simulink model "InductionMachine_dq"  (R2021b)
settings: Solver=FixedStepAuto  StartTime=0.0  StopTime=5  FixedStep=1e-3  RelTol=1e-3
values from neighbouring files (symbols this model uses):
  i_mr_0 = fl_rd_0 / L0    [InductionMachine_dq_cal.m]
  i_sd_0 = Isd_0    [InductionMachine_dq_cal.m]
  i_sq_0 = Isq_0    [InductionMachine_dq_cal.m]
  J = 0.2    [InductionMachine_cal.m]    (also in InductionMachine_dq_cal.m)
  L1 = 135.6e-3    (= 0.1356)    [InductionMachine_cal.m]    (also in InductionMachine_dq_cal.m)
  omega_m_0 = (2/P)*Wm    (= 188.495559215)    [InductionMachine_dq_cal.m]
  omega_vin = 120 * pi    (= 376.991118431)    [InductionMachine_dq_cal.m]
  P = 4    [InductionMachine_cal.m]    (also in InductionMachine_dq_cal.m)
  R1 = .75    (= 0.75)    [InductionMachine_cal.m]    (also in InductionMachine_dq_cal.m)
  sigma = 1 - (L0^2)/(L1*L2)    (= 0.0205423725864)    [InductionMachine_dq_cal.m]
  theta_0 = thetar    [InductionMachine_dq_cal.m]
  Tl = 0    [InductionMachine_cal.m]    (also in InductionMachine_dq_cal.m)
  Tr = L2/R2    (= 0.294782608696)    [InductionMachine_dq_cal.m]
  V_in = 163    [InductionMachine_dq_cal.m]
Description:
  | Lecture #20. page 138
  | Model of induction machine: Rotor Flux Oriented
  | Reference frame
settings Model: Creator=Dinh-Tuyen Le  LastModifiedBy=Dinh-Tuyen Le

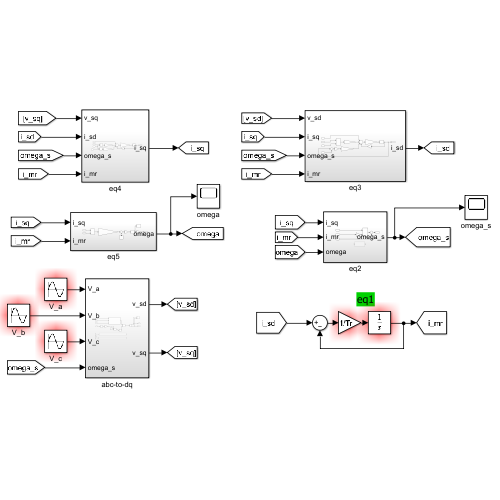
[thumbnail: Simulink's stored preview of the top-level diagram]
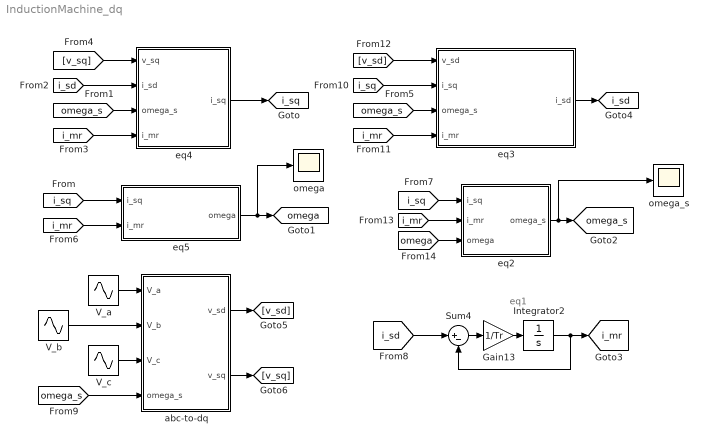
== system InductionMachine_dq ==
  note: eq1
  Gain13 : Gain  Gain=1/Tr
  Integrator2 : Integrator  InitialCondition=i_mr_0
  Sum4 : Sum  Inputs=|+-
  V_a : Sin  Amplitude=V_in  Frequency=omega_vin  Phase=pi/2  SampleTime=0
  V_b : Sin  Amplitude=V_in  Frequency=omega_vin  Phase=pi/2 -2 * pi / 3  SampleTime=0
  V_c : Sin  Amplitude=V_in  Frequency=omega_vin  Phase=pi/2 -4 * pi /3  SampleTime=0
  abc-to-dq : Subsystem
  eq2 : Subsystem
  eq3 : Subsystem
  eq4 : Subsystem
  eq5 : Subsystem
  omega : Scope
  omega_s : Scope
  tag scope: i_mr=global, i_sd=global, i_sq=global, omega=global, omega_s=global
  wires:
  [i_sd] -> Sum4/1
  Integrator2/1 -> Sum4/2, [i_mr]
  Sum4/1 -> Gain13/1
  Gain13/1 -> Integrator2/1
  V_a/1 -> abc-to-dq/1(V_a)
  V_b/1 -> abc-to-dq/2(V_b)
  V_c/1 -> abc-to-dq/3(V_c)
  [omega_s] -> abc-to-dq/4(omega_s)
  abc-to-dq/1(v_sd) -> [v_sd]
  abc-to-dq/2(v_sq) -> [v_sq]
  [i_sq] -> eq2/1(i_sq)
  [i_mr] -> eq2/2(i_mr)
  [omega] -> eq2/3(omega)
  eq2/1(omega_s) -> omega_s/1, [omega_s]
  [v_sd] -> eq3/1(v_sd)
  [i_sq] -> eq3/2(i_sq)
  [omega_s] -> eq3/3(omega_s)
  [i_mr] -> eq3/4(i_mr)
  eq3/1(i_sd) -> [i_sd]
  [i_sq] -> eq5/1(i_sq)
  [i_mr] -> eq5/2(i_mr)
  eq5/1(omega) -> omega/1, [omega]
  [v_sq] -> eq4/1(v_sq)
  [i_sd] -> eq4/2(i_sd)
  [omega_s] -> eq4/3(omega_s)
  [i_mr] -> eq4/4(i_mr)
  eq4/1(i_sq) -> [i_sq]

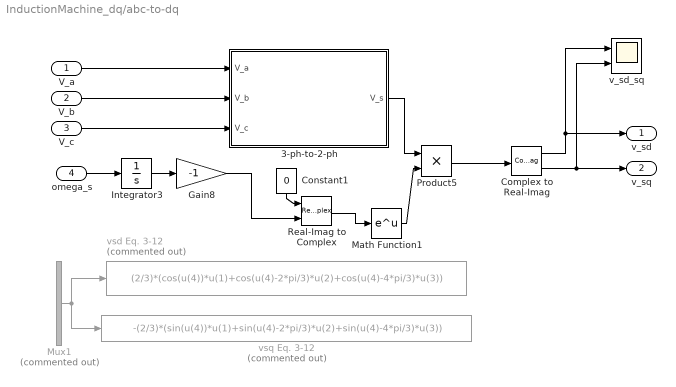
== system InductionMachine_dq/abc-to-dq ==
  V_a : Inport
  V_b : Inport  Port=2
  V_c : Inport  Port=3
  omega_s : Inport  Port=4
  3-ph-to-2-ph : Subsystem
  Complex to Real-Imag : ComplexToRealImag
  Constant1 : Constant  Value=0
  Gain8 : Gain  Gain=-1
  Integrator3 : Integrator  InitialCondition=theta_0
  Math Function1 : Math  OutputSignalType=complex  SaturateOnIntegerOverflow=on
  Mux1 : Mux  Commented=on
  Product5 : Product
  Real-Imag to Complex : RealImagToComplex
  v_sd_sq : Scope  NumInputPorts=2
  vsd Eq. 3-12 : Fcn  Commented=on  Expr=(2/3)*(cos(u(4))*u(1)+cos(u(4)-2*pi/3)*u(2)+cos(u(4)-4*pi/3)*u(3))
  vsq Eq. 3-12 : Fcn  Commented=on  Expr=-(2/3)*(sin(u(4))*u(1)+sin(u(4)-2*pi/3)*u(2)+sin(u(4)-4*pi/3)*u(3))
  v_sd : Outport
  v_sq : Outport  Port=2
  wires:
  3-ph-to-2-ph/1(V_s) -> Product5/1
  Math Function1/1 -> Product5/2
  Gain8/1 -> Real-Imag to Complex/2
  Constant1/1 -> Real-Imag to Complex/1
  Mux1/1 -> vsq Eq. 3-12/1, vsd Eq. 3-12/1
  Complex to Real-Imag/1 -> v_sd_sq/1, v_sd/1
  Real-Imag to Complex/1 -> Math Function1/1
  Integrator3/1 -> Gain8/1
  V_c/1 -> 3-ph-to-2-ph/3(V_c)
  V_b/1 -> 3-ph-to-2-ph/2(V_b)
  V_a/1 -> 3-ph-to-2-ph/1(V_a)
  omega_s/1 -> Integrator3/1
  Product5/1 -> Complex to Real-Imag/1
  Complex to Real-Imag/2 -> v_sd_sq/2, v_sq/1

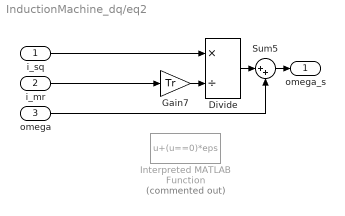
== system InductionMachine_dq/eq2 ==
  i_sq : Inport
  i_mr : Inport  Port=2
  omega : Inport  Port=3
  Divide : Product  Inputs=*/
  Gain7 : Gain  Gain=Tr
  Interpreted MATLAB Function : MATLABFcn  Commented=on  MATLABFcn=u+(u==0)*eps
  Sum5 : Sum  Inputs=|++
  omega_s : Outport
  wires:
  i_mr/1 -> Gain7/1
  Sum5/1 -> omega_s/1
  omega/1 -> Sum5/2
  Divide/1 -> Sum5/1
  i_sq/1 -> Divide/1
  Gain7/1 -> Divide/2

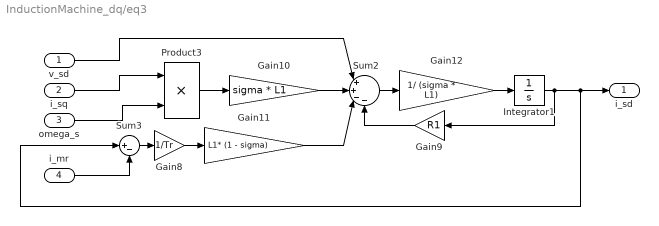
== system InductionMachine_dq/eq3 ==
  v_sd : Inport
  i_sq : Inport  Port=2
  omega_s : Inport  Port=3
  i_mr : Inport  Port=4
  Gain10 : Gain  Gain=sigma * L1
  Gain11 : Gain  Gain=L1* (1 - sigma)
  Gain12 : Gain  Gain=1/ (sigma * L1)
  Gain8 : Gain  Gain=1/Tr
  Gain9 : Gain  Gain=R1
  Integrator1 : Integrator  InitialCondition=i_sd_0
  Product3 : Product
  Sum2 : Sum  Inputs=|++--
  Sum3 : Sum  Inputs=|+-
  i_sd : Outport
  wires:
  Gain11/1 -> Sum2/3
  Sum2/1 -> Gain12/1
  i_mr/1 -> Sum3/2
  Product3/1 -> Gain10/1
  Gain10/1 -> Sum2/2
  v_sd/1 -> Sum2/1
  Integrator1/1 -> Sum3/1, i_sd/1, Gain9/1
  Gain9/1 -> Sum2/4
  Sum3/1 -> Gain8/1
  omega_s/1 -> Product3/2
  Gain8/1 -> Gain11/1
  i_sq/1 -> Product3/1
  Gain12/1 -> Integrator1/1

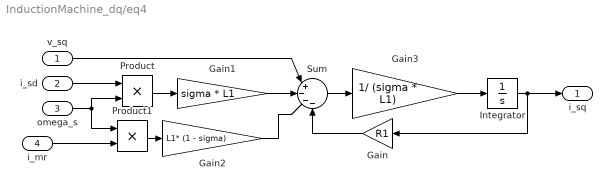
== system InductionMachine_dq/eq4 ==
  v_sq : Inport
  i_sd : Inport  Port=2
  omega_s : Inport  Port=3
  i_mr : Inport  Port=4
  Gain : Gain  Gain=R1
  Gain1 : Gain  Gain=sigma * L1
  Gain2 : Gain  Gain=L1* (1 - sigma)
  Gain3 : Gain  Gain=1/ (sigma * L1)
  Integrator : Integrator  InitialCondition=i_sq_0
  Product : Product
  Product1 : Product
  Sum : Sum  Inputs=|+---
  i_sq : Outport
  wires:
  Integrator/1 -> i_sq/1, Gain/1
  Gain1/1 -> Sum/2
  Sum/1 -> Gain3/1
  Gain3/1 -> Integrator/1
  omega_s/1 -> Product/2, Product1/1
  Gain/1 -> Sum/4
  Gain2/1 -> Sum/3
  Product1/1 -> Gain2/1
  Product/1 -> Gain1/1
  i_sd/1 -> Product/1
  v_sq/1 -> Sum/1
  i_mr/1 -> Product1/2

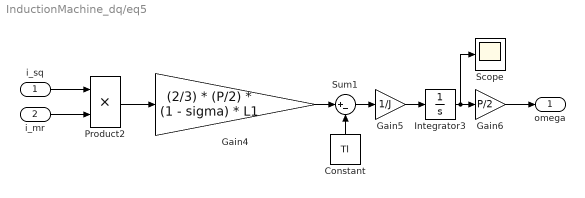
== system InductionMachine_dq/eq5 ==
  i_sq : Inport
  i_mr : Inport  Port=2
  Constant : Constant  Value=Tl
  Gain4 : Gain  Gain=(2/3) * (P/2) * (1 - sigma) * L1
  Gain5 : Gain  Gain=1/J
  Gain6 : Gain  Gain=P/2
  Integrator3 : Integrator  InitialCondition=omega_m_0
  Product2 : Product
  Scope : Scope
  Sum1 : Sum  Inputs=|+-
  omega : Outport
  wires:
  Product2/1 -> Gain4/1
  Gain4/1 -> Sum1/1
  Integrator3/1 -> Scope/1, Gain6/1
  Constant/1 -> Sum1/2
  i_sq/1 -> Product2/1
  Gain5/1 -> Integrator3/1
  Gain6/1 -> omega/1
  Sum1/1 -> Gain5/1
  i_mr/1 -> Product2/2

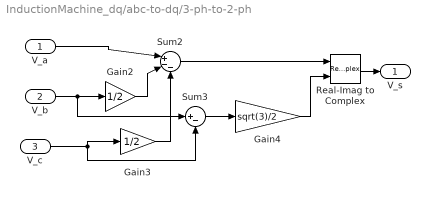
== system InductionMachine_dq/abc-to-dq/3-ph-to-2-ph ==
  V_a : Inport
  V_b : Inport  Port=2
  V_c : Inport  Port=3
  Gain2 : Gain  Gain=1/2
  Gain3 : Gain  Gain=1/2
  Gain4 : Gain  Gain=sqrt(3)/2
  Real-Imag to Complex : RealImagToComplex
  Sum2 : Sum  Inputs=|+--
  Sum3 : Sum  Inputs=|+-
  V_s : Outport
  wires:
  V_b/1 -> Sum3/1, Gain2/1
  Gain2/1 -> Sum2/2
  Gain4/1 -> Real-Imag to Complex/2
  Gain3/1 -> Sum2/3
  V_a/1 -> Sum2/1
  V_c/1 -> Sum3/2, Gain3/1
  Sum2/1 -> Real-Imag to Complex/1
  Sum3/1 -> Gain4/1
  Real-Imag to Complex/1 -> V_s/1
